simulink model "second_arm_compensation3"  (R2020b)
settings: Solver=ode15s  StartTime=0.0  StopTime=T  FixedStep=0.001  MaxStep=0.01  RelTol=1e-3
values from neighbouring files (symbols this model uses):
  a1A = 0.5    [sim_D_FB_J.m]
  a1B = 0.5    [sim_D_FB_J.m]
  a2A = 0.5    [sim_D_FB_J.m]
  a2B = 0.5    [sim_D_FB_J.m]
  a3A = 0.5    [sim_D_FB_J.m]
  a3B = 0.5    [sim_D_FB_J.m]
  dq0 = [0 0 0 0 0 0]'    [sim_second_arm_compensation.m]    (also in sim_second_arm_compensation3.m)
  friction = [fv1p fv2p fv1A fv2A fv3A fv1B fv2B fv3B]    [sim_second_arm_compensation.m]    (also in sim_second_arm_compensation2.m; sim_second_arm_compensation3.m)
  fv1A = 0    [sim_D_FB_J.m]
  fv1B = 0    [sim_D_FB_J.m]
  fv2A = 0    [sim_D_FB_J.m]
  fv2B = 0    [sim_D_FB_J.m]
  fv3A = 0    [sim_D_FB_J.m]
  fv3B = 0    [sim_D_FB_J.m]
  g = [0 -g0 0]'    [sim_second_arm_compensation.m]    (also in sim_second_arm_compensation2.m; sim_second_arm_compensation3.m)
  Gd_nullspace = 10*eye(6)    [sim_second_arm_compensation3.m]
  Gp_nullspace = 10*eye(6)    [sim_second_arm_compensation3.m]
  info = struct('n_joints', n_joints,                'n_links', n_links,                'n_ee', n_ee,                'current_frame_index',    [1  2 3 4 5 6 7  8 9 10],                'previous_frame_index',   [0  1 2 3 4 2 6  7 5  8],                'next_frame_index',       [2 36 4 5 9 7 8 10 0  0],                'next_frame_type',        [0  1 0 0 0 0 0  0 0  0],                'previous_joint_index',  ...(+449 chars)    [sim_second_arm_compensation.m]    (also in sim_second_arm_compensation2.m; sim_second_arm_compensation3.m)
  Kd = 5*eye(6)    [sim_D_FB_J.m]    (also in sim_second_arm_compensation.m; sim_second_arm_compensation2.m; sim_second_arm_compensation3.m = diag([5 5 5 1 1 1]))
  Kp = 5*eye(6)    [sim_D_FB_J.m]    (also in sim_second_arm_compensation.m; sim_second_arm_compensation2.m; sim_second_arm_compensation3.m = diag([5 5 5 1 1 1]))
  L = 3    [sim_D_FB_J.m]
  ml1A = 5    [sim_D_FB_J.m]
  ml1B = 5    [sim_D_FB_J.m]
  ml2A = 5    [sim_D_FB_J.m]
  ml2B = 5    [sim_D_FB_J.m]
  ml3A = 5    [sim_D_FB_J.m]
  ml3B = 5    [sim_D_FB_J.m]
  offA = -0.25    [sim_D_FB_J.m]
  offB = 0.25    [sim_D_FB_J.m]
  q0 = [th1A_0; th2A_0; th3A_0; th1B_0; th2B_0; th3B_0]    [sim_D_FB_J.m]    (also in sim_second_arm_compensation.m; sim_second_arm_compensation2.m; sim_second_arm_compensation3.m)
  th1A_0 = -pi/2    (= -1.57079632679)    [sim_D_FB_J.m]    (also in sim_second_arm_compensation.m = 0; sim_second_arm_compensation2.m = 0; sim_second_arm_compensation3.m = -0.523598775598)
  th1B_0 = -pi/2    (= -1.57079632679)    [sim_D_FB_J.m]    (also in sim_second_arm_compensation.m = 0; sim_second_arm_compensation2.m = 0; sim_second_arm_compensation3.m = 0.523598775598)
  th2A_0 = -pi/8    (= -0.392699081699)    [sim_D_FB_J.m]    (also in sim_second_arm_compensation.m; sim_second_arm_compensation2.m; sim_second_arm_compensation3.m = 0.523598775598)
  th2B_0 = pi/8    (= 0.392699081699)    [sim_D_FB_J.m]    (also in sim_second_arm_compensation.m; sim_second_arm_compensation2.m; sim_second_arm_compensation3.m = -0.523598775598)
  th3A_0 = -pi/8    (= -0.392699081699)    [sim_D_FB_J.m]    (also in sim_second_arm_compensation.m; sim_second_arm_compensation2.m; sim_second_arm_compensation3.m = 0.523598775598)
  th3B_0 = pi/8    (= 0.392699081699)    [sim_D_FB_J.m]    (also in sim_second_arm_compensation.m; sim_second_arm_compensation2.m; sim_second_arm_compensation3.m = -0.523598775598)
undefined symbols (not defined in the file or in its folder): D, l1A, l1B, l2A, l2B, l3A, l3B, m_cables, m_crane, m_platform, X, Y, Z
libraries: sm_lib x137, nesl_utility x31
(part 4 of 4)

== matlab function second_arm_compensation3/CLIK 2/Controller ==
  data: in input; q input; qd input; a1A parameter; a2A parameter; a3A parameter; a1B parameter; a2B parameter; a3B parameter; y output; offA parameter; offB parameter; ml1A parameter; ml2A parameter; ml3A parameter; ml1B parameter; ml2B parameter; ml3B parameter; l1A parameter; l2A parameter; l3A parameter; l1B parameter; l2B parameter; l3B parameter; Gd_nullspace parameter; Gp_nullspace parameter; q0 parameter
function y  = fcn(in, q, qd, ...
                  a1A, a2A, a3A, a1B, a2B, a3B, offA, offB, ...
                  ml1A, ml2A, ml3A, ml1B, ml2B, ml3B, ...
                  l1A, l2A, l3A, l1B, l2B, l3B, Gd_nullspace, Gp_nullspace, q0)

% Input
th1A = q(1);
th2A = q(2);
th3A = q(3);
th1B = q(4);
th2B = q(5);
th3B = q(6);

% Jacobiano
Ja = [                                                                                                     a2A*cos(th1A + th2A) + a1A*cos(th1A) + a3A*cos(th1A + th2A + th3A),                                                               a2A*cos(th1A + th2A) + a3A*cos(th1A + th2A + th3A),                                 a3A*cos(th1A + th2A + th3A),                                                                                                                                                                       0,                                                                                                                0,                                                           0;
                                                                                                           a2A*sin(th1A + th2A) + a1A*sin(th1A) + a3A*sin(th1A + th2A + th3A),                                                               a2A*sin(th1A + th2A) + a3A*sin(th1A + th2A + th3A),                                 a3A*sin(th1A + th2A + th3A),                                                                                                                                                                       0,                                                                                                                0,                                                           0;
                                                                                                                                                                            1,                                                                                                                1,                                                           1,                                                                                                                                                                       0,                                                                                                                0,                                                           0;      
                                                                                                                                                                            0,                                                                                                                0,                                                           0,                                                                                                      a2B*cos(th1B + th2B) + a1B*cos(th1B) + a3B*cos(th1B + th2B + th3B),                                                               a2B*cos(th1B + th2B) + a3B*cos(th1B + th2B + th3B),                                 a3B*cos(th1B + th2B + th3B);
                                                                                                                                                                            0,                                                                                                                0,                                                           0,                                                                                                      a2B*sin(th1B + th2B) + a1B*sin(th1B) + a3B*sin(th1B + th2B + th3B),                                                               a2B*sin(th1B + th2B) + a3B*sin(th1B + th2B + th3B),                                 a3B*sin(th1B + th2B + th3B);
      (ml3A*(a2A*cos(th1A + th2A) + a1A*cos(th1A) + l3A*cos(th1A + th2A + th3A)) + ml2A*(l2A*cos(th1A + th2A) + a1A*cos(th1A)) + l1A*ml1A*cos(th1A))/(2*(ml1A + ml2A + ml3A)), (ml3A*(a2A*cos(th1A + th2A) + l3A*cos(th1A + th2A + th3A)) + l2A*ml2A*cos(th1A + th2A))/(2*(ml1A + ml2A + ml3A)), (l3A*ml3A*cos(th1A + th2A + th3A))/(2*(ml1A + ml2A + ml3A)), (ml3B*(a2B*cos(th1B + th2B) + a1B*cos(th1B) + l3B*cos(th1B + th2B + th3B)) + ml2B*(l2B*cos(th1B + th2B) + a1B*cos(th1B)) + l1B*ml1B*cos(th1B))/(2*(ml1B + ml2B + ml3B)), (ml3B*(a2B*cos(th1B + th2B) + l3B*cos(th1B + th2B + th3B)) + l2B*ml2B*cos(th1B + th2B))/(2*(ml1B + ml2B + ml3B)), (l3B*ml3B*cos(th1B + th2B + th3B))/(2*(ml1B + ml2B + ml3B))];

% Control
y = pinv(Ja)*in + (eye(6)-pinv(Ja)*Ja)*(Gd_nullspace*(-qd)+Gp_nullspace*(q0-q));

end

== matlab function second_arm_compensation3/MATLAB Function ==
  data: theta input; peA output; peB output; oA output; oB output
function [peA,peB,oA,oB] = fcn(theta)

n_joints = 8;

L = 3.16 + 0.126;           % [m] (Distance between the first passive joint and the second passive joint)
D = 1.047;                  % [m] (Distance between the second passive joint and the base of the schunks)
L1 = 0.350;                 % [m] (Distance between the center of the two ERB145)
L2 = 0.305;                 % [m] (Distance between the center of the second ERB145 and the ERB115)
L3 = 0.2662;                % [m] (Distance between the center of the ERB115 and the end-effector (center of the tip of the finger of the gripper))
offA = -0.19;               % [m] (Half of the distance between the arms)
offB = 0.19;                % [m] (Half of the distance between the arms)
a1A = L1;
a2A = L2;
a3A = L3;
a1B = L1;
a2B = L2;
a3B = L3;
l1A = a1A/2;
l2A = a2A/2;
l3A = a3A/2;
l1B = a1B/2;
l2B = a2B/2;
l3B = a3B/2;
    
% Initializations
SA = zeros(6,6);
SB = zeros(6,6);

% Kinematic parameters
omega1 = [0 0 1]';
omega2 = [0 0 1]';
omega1A = [0 0 1]';
omega2A = [0 0 1]';
omega3A = [0 0 1]';
omega1B = [0 0 1]';
omega2B = [0 0 1]';
omega3B = [0 0 1]';
q1 = [0 0 0]';
q2 = [0 -L 0]';
q1A = [offA -L-D 0]';
q2A = [offA -L-D-a1A 0]';
q3A = [offA -L-D-a1A-a2A 0]';
q1B = [offB -L-D 0]';
q2B = [offB -L-D-a1B 0]';
q3B = [offB -L-D-a1B-a2B 0]';



% Computation M_{b,i}
M1 = [ 0  1  0  0; 
      -1  0  0  0;
       0  0  1  0
       0  0  0  1];

M2 = [ 1  0  0  0; 
       0  1  0 -L;
       0  0  1  0
       0  0  0  1];

M1A = [ 0  1  0   offA; 
       -1  0  0   -L-D;
        0  0  1    0
        0  0  0    1];

M2A = [ 0  1  0   offA; 
       -1  0  0 -L-D-a1A;
        0  0  1    0
        0  0  0    1];
   
M3A = [ 0  1  0   offA; 
       -1  0  0 -L-D-a1A-a2A;
        0  0  1    0
        0  0  0    1];

M1B = [ 0  1  0   offB; 
        -1  0  0 -L-D-l1B;
         0  0  1    0
         0  0  0    1];

M2B = [ 0  1  0   offB; 
        -1  0  0 -L-D-a1B-l2B;
         0  0  1    0
         0  0  0    1];
   
M3B = [ 0  1  0   offB; 
        -1  0  0 -L-D-a1B-a2B-l3B;
         0  0  1    0
         0  0  0    1];

MeA = [ 0  1  0   offA; 
        -1  0  0 -L-D-a1A-a2A-a3A;
         0  0  1    0
         0  0  0    1];

MeB = [ 0  1  0   offB; 
         -1  0  0 -L-D-a1B-a2B-a3B;
          0  0  1    0
          0  0  0    1];


% Screw axis computation
omegaA = [omega1, omega2, omega1A, omega2A, omega3A];
qA = [q1, q2, q1A, q2A, q3A];
for i = 1:length(omegaA)
    vA = cross(-omegaA(:,i),qA(:,i));
    SA(:,i) = [omegaA(:,i); vA];
end
omegaB = [omega1, omega2, omega1B, omega2B, omega3B];
qB = [q1, q2, q1B, q2B, q3B];
for i = 1:length(omegaB)
    vB = cross(-omegaB(:,i),qB(:,i));
    SB(:,i) = [omegaB(:,i); vB];
end

    
% Kinematics (position of the joints and of the end effector)
TeA = fkin_f(theta(1:5), 5, MeA, SA(:,1:5));
TeB = fkin_f([theta(1:2); theta(6:8)], 5, MeB, SB(:,1:5));

peA = TeA(1:2,4);
peB = TeB(1:2,4);
oA = rotm2eul(TeA(1:3,1:3));
oB = rotm2eul(TeB(1:3,1:3));

end

== matlab function second_arm_compensation3/CLIK 2/Direct Kinematics ==
  data: q input; xe output; a1A parameter; a2A parameter; a3A parameter; a1B parameter; a2B parameter; a3B parameter; offA parameter; offB parameter; ml1A parameter; ml2A parameter; ml3A parameter; ml1B parameter; ml2B parameter; ml3B parameter; l1A parameter; l2A parameter; l3A parameter; l1B parameter; l2B parameter; l3B parameter
function xe = fcn(q, ...
                  a1A, a2A, a3A, a1B, a2B, a3B, offA, offB, ...
                  ml1A, ml2A, ml3A, ml1B, ml2B, ml3B, ...
                  l1A, l2A, l3A, l1B, l2B, l3B)

% Input
th1A = q(1);
th2A = q(2);
th3A = q(3);
th1B = q(4);
th2B = q(5);
th3B = q(6);
       
% Center of Mass of the arms
pl1A = [offA+l1A*sin(th1A), -l1A*cos(th1A)]';
pl2A = [offA+a1A*sin(th1A)+l2A*sin(th1A+th2A), -a1A*cos(th1A)-l2A*cos(th1A+th2A)]';
pl3A = [offA+a1A*sin(th1A)+a2A*sin(th1A+th2A)+l3A*sin(th1A+th2A+th3A), -a1A*cos(th1A)-a2A*cos(th1A+th2A)-l3A*cos(th1A+th2A+th3A)]';
pl1B = [offB+l1B*sin(th1B), -l1B*cos(th1B)]';
pl2B = [offB+a1B*sin(th1B)+l2B*sin(th1B+th2B), -a1B*cos(th1B)-l2B*cos(th1B+th2B)]';
pl3B = [offB+a1B*sin(th1B)+a2B*sin(th1B+th2B)+l3B*sin(th1B+th2B+th3B), -a1B*cos(th1B)-a2B*cos(th1B+th2B)-l3B*cos(th1B+th2B+th3B)]';

cmxA = (ml1A*pl1A(1)+ml2A*pl2A(1)+ml3A*pl3A(1))/(ml1A+ml2A+ml3A);
cmyA = (ml1A*pl1A(2)+ml2A*pl2A(2)+ml3A*pl3A(2))/(ml1A+ml2A+ml3A);
cmxB = (ml1B*pl1B(1)+ml2B*pl2B(1)+ml3B*pl3B(1))/(ml1B+ml2B+ml3B);
cmyB = (ml1B*pl1B(2)+ml2B*pl2B(2)+ml3B*pl3B(2))/(ml2B+ml2B+ml3B);
cmx = (cmxA + cmxB)/2;

% Cinematica diretta
xe = [ offA + a1A*sin(th1A) + a2A*sin(th1A + th2A) + a3A*sin(th1A + th2A + th3A);
            - a1A*cos(th1A) - a2A*cos(th1A + th2A) - a3A*cos(th1A + th2A + th3A);
                                                              th1A + th2A + th3A;
       offB + a1B*sin(th1B) + a2B*sin(th1B + th2B) + a3B*sin(th1B + th2B + th3B);
            - a1B*cos(th1B) - a2B*cos(th1B + th2B) - a3B*cos(th1B + th2B + th3B);
                                                                            cmx];

end

== matlab function second_arm_compensation3/CLIK 2/Ja*qd ==
  data: q input; qd input; xe_dot output; a1A parameter; a2A parameter; a3A parameter; a1B parameter; a2B parameter; a3B parameter; offA parameter; offB parameter; ml1A parameter; ml2A parameter; ml3A parameter; ml1B parameter; ml2B parameter; ml3B parameter; l1A parameter; l2A parameter; l3A parameter; l1B parameter; l2B parameter; l3B parameter
function xe_dot = fcn(q, qd, ...
                      a1A, a2A, a3A, a1B, a2B, a3B, offA, offB, ...
                      ml1A, ml2A, ml3A, ml1B, ml2B, ml3B, ...
                      l1A, l2A, l3A, l1B, l2B, l3B)

% Input
th1A = q(1);
th2A = q(2);
th3A = q(3);
th1B = q(4);
th2B = q(5);
th3B = q(6);

Ja = [                                                                                                     a2A*cos(th1A + th2A) + a1A*cos(th1A) + a3A*cos(th1A + th2A + th3A),                                                               a2A*cos(th1A + th2A) + a3A*cos(th1A + th2A + th3A),                                 a3A*cos(th1A + th2A + th3A),                                                                                                                                                                       0,                                                                                                                0,                                                           0;
                                                                                                           a2A*sin(th1A + th2A) + a1A*sin(th1A) + a3A*sin(th1A + th2A + th3A),                                                               a2A*sin(th1A + th2A) + a3A*sin(th1A + th2A + th3A),                                 a3A*sin(th1A + th2A + th3A),                                                                                                                                                                       0,                                                                                                                0,                                                           0;
                                                                                                                                                                            1,                                                                                                                1,                                                           1,                                                                                                                                                                       0,                                                                                                                0,                                                           0;      
                                                                                                                                                                            0,                                                                                                                0,                                                           0,                                                                                                      a2B*cos(th1B + th2B) + a1B*cos(th1B) + a3B*cos(th1B + th2B + th3B),                                                               a2B*cos(th1B + th2B) + a3B*cos(th1B + th2B + th3B),                                 a3B*cos(th1B + th2B + th3B);
                                                                                                                                                                            0,                                                                                                                0,                                                           0,                                                                                                      a2B*sin(th1B + th2B) + a1B*sin(th1B) + a3B*sin(th1B + th2B + th3B),                                                               a2B*sin(th1B + th2B) + a3B*sin(th1B + th2B + th3B),                                 a3B*sin(th1B + th2B + th3B);
      (ml3A*(a2A*cos(th1A + th2A) + a1A*cos(th1A) + l3A*cos(th1A + th2A + th3A)) + ml2A*(l2A*cos(th1A + th2A) + a1A*cos(th1A)) + l1A*ml1A*cos(th1A))/(2*(ml1A + ml2A + ml3A)), (ml3A*(a2A*cos(th1A + th2A) + l3A*cos(th1A + th2A + th3A)) + l2A*ml2A*cos(th1A + th2A))/(2*(ml1A + ml2A + ml3A)), (l3A*ml3A*cos(th1A + th2A + th3A))/(2*(ml1A + ml2A + ml3A)), (ml3B*(a2B*cos(th1B + th2B) + a1B*cos(th1B) + l3B*cos(th1B + th2B + th3B)) + ml2B*(l2B*cos(th1B + th2B) + a1B*cos(th1B)) + l1B*ml1B*cos(th1B))/(2*(ml1B + ml2B + ml3B)), (ml3B*(a2B*cos(th1B + th2B) + l3B*cos(th1B + th2B + th3B)) + l2B*ml2B*cos(th1B + th2B))/(2*(ml1B + ml2B + ml3B)), (l3B*ml3B*cos(th1B + th2B + th3B))/(2*(ml1B + ml2B + ml3B))];

xe_dot = Ja*qd;

end

== matlab function second_arm_compensation3/CLIK 2/Ja_dot*qd ==
  data: q input; qd input; out output; a1A parameter; a2A parameter; a3A parameter; a1B parameter; a2B parameter; a3B parameter; offA parameter; offB parameter; ml1A parameter; ml2A parameter; ml3A parameter; ml1B parameter; ml2B parameter; ml3B parameter; l1A parameter; l2A parameter; l3A parameter; l1B parameter; l2B parameter; l3B parameter
function out = fcn(q, qd, ...
                  a1A, a2A, a3A, a1B, a2B, a3B, offA, offB, ...
                  ml1A, ml2A, ml3A, ml1B, ml2B, ml3B, ...
                  l1A, l2A, l3A, l1B, l2B, l3B)

% Input
th1A = q(1);
th2A = q(2);
th3A = q(3);
th1B = q(4);
th2B = q(5);
th3B = q(6);
dth1A = qd(1);
dth2A = qd(2);
dth3A = qd(3);
dth1B = qd(4);
dth2B = qd(5);
dth3B = qd(6);

% Derivata dello Jacobiano
Jad = [                                                                                                                                  - a1A*dth1A*sin(th1A) - a3A*sin(th1A + th2A + th3A)*(dth1A + dth2A + dth3A) - a2A*sin(th1A + th2A)*(dth1A + dth2A),                                                                                - a3A*sin(th1A + th2A + th3A)*(dth1A + dth2A + dth3A) - a2A*sin(th1A + th2A)*(dth1A + dth2A),                                   -a3A*sin(th1A + th2A + th3A)*(dth1A + dth2A + dth3A),                                                                                                                                                                                                                                                    0,                                                                                                                                                                           0,                                                                                      0;
                                                                                                                                           a3A*cos(th1A + th2A + th3A)*(dth1A + dth2A + dth3A) + a2A*cos(th1A + th2A)*(dth1A + dth2A) + a1A*dth1A*cos(th1A),                                                                                  a3A*cos(th1A + th2A + th3A)*(dth1A + dth2A + dth3A) + a2A*cos(th1A + th2A)*(dth1A + dth2A),                                    a3A*cos(th1A + th2A + th3A)*(dth1A + dth2A + dth3A),                                                                                                                                                                                                                                                    0,                                                                                                                                                                           0,                                                                                      0;
                                                                                                                                                                                                                                                          0,                                                                                                                                                                           0,                                                                                      0,                                                                                                                                                                                                                                                    0,                                                                                                                                                                           0,                                                                                      0;
                                                                                                                                                                                                                                                          0,                                                                                                                                                                           0,                                                                                      0,                                                                                                                                   - a1B*dth1B*sin(th1B) - a3B*sin(th1B + th2B + th3B)*(dth1B + dth2B + dth3B) - a2B*sin(th1B + th2B)*(dth1B + dth2B),                                                                                - a3B*sin(th1B + th2B + th3B)*(dth1B + dth2B + dth3B) - a2B*sin(th1B + th2B)*(dth1B + dth2B),                                   -a3B*sin(th1B + th2B + th3B)*(dth1B + dth2B + dth3B);
                                                                                                                                                                                                                                                          0,                                                                                                                                                                           0,                                                                                      0,                                                                                                                                     a3B*cos(th1B + th2B + th3B)*(dth1B + dth2B + dth3B) + a2B*cos(th1B + th2B)*(dth1B + dth2B) + a1B*dth1B*cos(th1B),                                                                                  a3B*cos(th1B + th2B + th3B)*(dth1B + dth2B + dth3B) + a2B*cos(th1B + th2B)*(dth1B + dth2B),                                    a3B*cos(th1B + th2B + th3B)*(dth1B + dth2B + dth3B);
       -(ml3A*(a1A*dth1A*sin(th1A) + l3A*sin(th1A + th2A + th3A)*(dth1A + dth2A + dth3A) + a2A*sin(th1A + th2A)*(dth1A + dth2A)) + ml2A*(a1A*dth1A*sin(th1A) + l2A*sin(th1A + th2A)*(dth1A + dth2A)) + dth1A*l1A*ml1A*sin(th1A))/(2*ml1A + 2*ml2A + 2*ml3A), -(ml3A*(l3A*sin(th1A + th2A + th3A)*(dth1A + dth2A + dth3A) + a2A*sin(th1A + th2A)*(dth1A + dth2A)) + l2A*ml2A*sin(th1A + th2A)*(dth1A + dth2A))/(2*ml1A + 2*ml2A + 2*ml3A), -(l3A*ml3A*sin(th1A + th2A + th3A)*(dth1A + dth2A + dth3A))/(2*ml1A + 2*ml2A + 2*ml3A), -(ml3B*(a1B*dth1B*sin(th1B) + l3B*sin(th1B + th2B + th3B)*(dth1B + dth2B + dth3B) + a2B*sin(th1B + th2B)*(dth1B + dth2B)) + ml2B*(a1B*dth1B*sin(th1B) + l2B*sin(th1B + th2B)*(dth1B + dth2B)) + dth1B*l1B*ml1B*sin(th1B))/(2*ml1B + 2*ml2B + 2*ml3B), -(ml3B*(l3B*sin(th1B + th2B + th3B)*(dth1B + dth2B + dth3B) + a2B*sin(th1B + th2B)*(dth1B + dth2B)) + l2B*ml2B*sin(th1B + th2B)*(dth1B + dth2B))/(2*ml1B + 2*ml2B + 2*ml3B), -(l3B*ml3B*sin(th1B + th2B + th3B)*(dth1B + dth2B + dth3B))/(2*ml1B + 2*ml2B + 2*ml3B)];

out = Jad*qd;

end

== matlab function second_arm_compensation3/CLIK 1/Controller ==
  data: in input; q input; qd input; a1A parameter; a2A parameter; a3A parameter; a1B parameter; a2B parameter; a3B parameter; y output; offA parameter; offB parameter; Gd_nullspace parameter; Gp_nullspace parameter; q0 parameter
function y  = fcn(in, q, qd, ...
                  a1A, a2A, a3A, a1B, a2B, a3B, offA, offB, ...
                  Gd_nullspace, Gp_nullspace, q0)

% Input
th1A = q(1);
th2A = q(2);
th3A = q(3);
th1B = q(4);
th2B = q(5);
th3B = q(6);

% Jacobiano
Ja = [a2A*cos(th1A + th2A) + a1A*cos(th1A) + a3A*cos(th1A + th2A + th3A), a2A*cos(th1A + th2A) + a3A*cos(th1A + th2A + th3A), a3A*cos(th1A + th2A + th3A),                                                                  0,                                                  0,                           0;
      a2A*sin(th1A + th2A) + a1A*sin(th1A) + a3A*sin(th1A + th2A + th3A), a2A*sin(th1A + th2A) + a3A*sin(th1A + th2A + th3A), a3A*sin(th1A + th2A + th3A),                                                                  0,                                                  0,                           0;
                                                                       1,                                                  1,                           1,                                                                  0,                                                  0,                           0;
                                                                       0,                                                  0,                           0, a2B*cos(th1B + th2B) + a1B*cos(th1B) + a3B*cos(th1B + th2B + th3B), a2B*cos(th1B + th2B) + a3B*cos(th1B + th2B + th3B), a3B*cos(th1B + th2B + th3B);
                                                                       0,                                                  0,                           0, a2B*sin(th1B + th2B) + a1B*sin(th1B) + a3B*sin(th1B + th2B + th3B), a2B*sin(th1B + th2B) + a3B*sin(th1B + th2B + th3B), a3B*sin(th1B + th2B + th3B);
                                                                       0,                                                  0,                           0,                                                                  1,                                                  1,                           1];

% Control
y = pinv(Ja)*in + (eye(6)-pinv(Ja)*Ja)*(Gd_nullspace*(-qd)+Gp_nullspace*(q0-q));

end
